simulink model "untitled"  (R2020a)
settings: Solver=VariableStepAuto  StartTime=0.0  StopTime=10.0  RelTol=1e-3
settings Model: Creator=mdc8965  LastModifiedBy=mdc8965

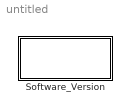
== system untitled ==
  Software_Version : Subsystem  RequirementInfo={} %GIDa_286d241e_ef8a_4a4c_bee6_909e0a809aac

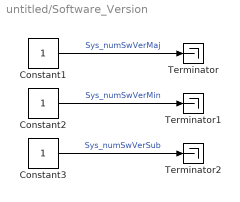
== system untitled/Software_Version ==
  Constant1 : Constant  RequirementInfo={} %GIDa_d4b1a489_3363_4e31_8078_a1e7a7e23799  OutDataTypeStr=uint8
  Constant2 : Constant  RequirementInfo={} %GIDa_d8d35667_c48c_409a_b7f9_dd424d45dccb  OutDataTypeStr=uint8
  Constant3 : Constant  RequirementInfo={} %GIDa_9ff88862_4d5a_4c72_aaec_0ff05df10fd4  OutDataTypeStr=uint8
  Terminator : Terminator
      settings: RequirementInfo={} %GIDa_6971c628_d7a3_4239_bb4a_b1daa5b90e41
  Terminator1 : Terminator
      settings: RequirementInfo={} %GIDa_96d7e49a_bfa9_47b3_a4cd_3b15877c8214
  Terminator2 : Terminator
      settings: RequirementInfo={} %GIDa_9a2888b6_ac41_4433_b9c3_f61bdf0b7a4c
  wires:
  Constant1/1 -> Terminator/1  "Sys_numSwVerMaj"
  Constant2/1 -> Terminator1/1  "Sys_numSwVerMin"
  Constant3/1 -> Terminator2/1  "Sys_numSwVerSub"
